simulink model "OPENXWD"  (R2021b)
settings: Solver=ode45  StartTime=0.0  StopTime=inf  RelTol=1e-3  EnableMultiTasking=on
PreLoadFcn:
  | run('Parameters\FSE_Parameters.m')
undefined symbols (not defined in the file): i_Diff
libraries: simulink x28, CarMaker4SL x17, eeGeneralControl x6
(part 2 of 8)

== system OPENXWD/CarMaker/IPG Vehicle/CarAndTrailer/Forces/Tires ==
  note: The TireXX_Out signals will only be used if FileIdent is "CarMaker-Tire-CM4SL" in the tire parameter file!
      | An example parameter file can be found in Data/Tire/DT_CM4SL_UserTire.
  Sync_In : Inport
  TireFL_In : Inport  Port=2
  TireFR_In : Inport  Port=3
  TireRL_In : Inport  Port=4
  TireRR_In : Inport  Port=5
  Bus Creator{1..4} (4 alike) : BusCreator  Inputs=11
  Demux{1..3,8} (4 alike) : Demux  Outputs=7
      settings: DisplayOption=none
  TireFL : Subsystem
  TireFR : Subsystem
  TireRL : Subsystem
  TireRR : Subsystem
  TireFL_Out : Outport
  TireFR_Out : Outport  Port=2
  TireRL_Out : Outport  Port=3
  TireRR_Out : Outport  Port=4
  wires:
  Sync_In/1 -> TireRR/1(Sync_In), TireRL/1(Sync_In), TireFR/1(Sync_In), TireFL/1(Sync_In)
  Bus Creator4/1 -> TireRR_Out/1
  Bus Creator2/1 -> TireRL_Out/1
  Bus Creator1/1 -> TireFR_Out/1
  Demux3/5 -> TireRR/6(Rim_turnv)  "Tire_In Rim_turnv"
  Demux3/4 -> TireRR/5(Rim_rotv)  "Tire_In Rim_rotv"
  Demux3/1 -> TireRR/2(Load)  "Tire_In Load"
  Demux3/7 -> TireRR/8(muRoad)  "Tire_In mu"
  Demux3/6 -> TireRR/7(InclinAngle)  "Tire_In Camber"
  Demux3/2 -> TireRR/3(vxtrans)  "Tire_In vxtrans"
  Demux3/3 -> TireRR/4(vytrans)  "Tire_In vytrans"
  TireRR/11(AlignTrq) -> Bus Creator4/11  "Tire_Out AlignTrq"
  TireRR/10(RollResist) -> Bus Creator4/10  "Tire_Out RollResist"
  TireRR/9(OverturnTrq) -> Bus Creator4/9  "Tire_Out OverturnTrq"
  TireRR/8(LoadFrc) -> Bus Creator4/8  "Tire_Out LoadFrc"
  TireRR/7(SideFrc) -> Bus Creator4/7  "Tire_Out SideFrc"
  TireRR/6(LongFrc) -> Bus Creator4/6  "Tire_Out LongFrc"
  TireRR/5(vBelt) -> Bus Creator4/5  "Tire_Out vBelt"
  TireRR/4(rBelt_eff) -> Bus Creator4/4  "Tire_Out rBelt_eff"
  TireRR/3(TurnSlp) -> Bus Creator4/3  "Tire_Out TurnSlp"
  TireRR/1(Slp) -> Bus Creator4/1  "Tire_Out Slp"
  TireRR/2(Alpha) -> Bus Creator4/2  "Tire_Out Alpha"
  Demux2/5 -> TireRL/6(Rim_turnv)  "Tire_In Rim_turnv"
  Demux2/4 -> TireRL/5(Rim_rotv)  "Tire_In Rim_rotv"
  Demux2/1 -> TireRL/2(Load)  "Tire_In Load"
  Demux2/7 -> TireRL/8(muRoad)  "Tire_In mu"
  Demux2/6 -> TireRL/7(InclinAngle)  "Tire_In Camber"
  Demux2/2 -> TireRL/3(vxtrans)  "Tire_In vxtrans"
  Demux2/3 -> TireRL/4(vytrans)  "Tire_In vytrans"
  TireRL/11(AlignTrq) -> Bus Creator2/11  "Tire_Out AlignTrq"
  TireRL/10(RollResist) -> Bus Creator2/10  "Tire_Out RollResist"
  TireRL/9(OverturnTrq) -> Bus Creator2/9  "Tire_Out OverturnTrq"
  TireRL/8(LoadFrc) -> Bus Creator2/8  "Tire_Out LoadFrc"
  TireRL/7(SideFrc) -> Bus Creator2/7  "Tire_Out SideFrc"
  TireRL/6(LongFrc) -> Bus Creator2/6  "Tire_Out LongFrc"
  TireRL/5(vBelt) -> Bus Creator2/5  "Tire_Out vBelt"
  TireRL/4(rBelt_eff) -> Bus Creator2/4  "Tire_Out rBelt_eff"
  TireRL/3(TurnSlp) -> Bus Creator2/3  "Tire_Out TurnSlp"
  TireRL/1(Slp) -> Bus Creator2/1  "Tire_Out Slp"
  TireRL/2(Alpha) -> Bus Creator2/2  "Tire_Out Alpha"
  Demux1/5 -> TireFR/6(Rim_turnv)  "Tire_In Rim_turnv"
  Demux1/4 -> TireFR/5(Rim_rotv)  "Tire_In Rim_rotv"
  Demux1/1 -> TireFR/2(Load)  "Tire_In Load"
  Demux1/7 -> TireFR/8(muRoad)  "Tire_In mu"
  Demux1/6 -> TireFR/7(InclinAngle)  "Tire_In Camber"
  Demux1/2 -> TireFR/3(vxtrans)  "Tire_In vxtrans"
  Demux1/3 -> TireFR/4(vytrans)  "Tire_In vytrans"
  TireFR/11(AlignTrq) -> Bus Creator1/11  "Tire_Out AlignTrq"
  TireFR/10(RollResist) -> Bus Creator1/10  "Tire_Out RollResist"
  TireFR/9(OverturnTrq) -> Bus Creator1/9  "Tire_Out OverturnTrq"
  TireFR/8(LoadFrc) -> Bus Creator1/8  "Tire_Out LoadFrc"
  TireFR/7(SideFrc) -> Bus Creator1/7  "Tire_Out SideFrc"
  TireFR/6(LongFrc) -> Bus Creator1/6  "Tire_Out LongFrc"
  TireFR/5(vBelt) -> Bus Creator1/5  "Tire_Out vBelt"
  TireFR/4(rBelt_eff) -> Bus Creator1/4  "Tire_Out rBelt_eff"
  TireFR/3(TurnSlp) -> Bus Creator1/3  "Tire_Out TurnSlp"
  TireFR/1(Slp) -> Bus Creator1/1  "Tire_Out Slp"
  TireFR/2(Alpha) -> Bus Creator1/2  "Tire_Out Alpha"
  Demux8/5 -> TireFL/6(Rim_turnv)  "Tire_In Rim_turnv"
  Demux8/4 -> TireFL/5(Rim_rotv)  "Tire_In Rim_rotv"
  TireFL_In/1 -> Demux8/1
  Demux8/1 -> TireFL/2(Load)  "Tire_In Load"
  Demux8/7 -> TireFL/8(muRoad)  "Tire_In mu"
  Demux8/6 -> TireFL/7(InclinAngle)  "Tire_In Camber"
  Demux8/2 -> TireFL/3(vxtrans)  "Tire_In vxtrans"
  Demux8/3 -> TireFL/4(vytrans)  "Tire_In vytrans"
  TireFL/11(AlignTrq) -> Bus Creator3/11  "Tire_Out AlignTrq"
  TireFL/10(RollResist) -> Bus Creator3/10  "Tire_Out RollResist"
  TireFL/9(OverturnTrq) -> Bus Creator3/9  "Tire_Out OverturnTrq"
  TireFL/8(LoadFrc) -> Bus Creator3/8  "Tire_Out LoadFrc"
  TireFL/7(SideFrc) -> Bus Creator3/7  "Tire_Out SideFrc"
  TireFL/6(LongFrc) -> Bus Creator3/6  "Tire_Out LongFrc"
  TireFL/5(vBelt) -> Bus Creator3/5  "Tire_Out vBelt"
  TireFL/4(rBelt_eff) -> Bus Creator3/4  "Tire_Out rBelt_eff"
  TireFL/3(TurnSlp) -> Bus Creator3/3  "Tire_Out TurnSlp"
  TireFL/1(Slp) -> Bus Creator3/1  "Tire_Out Slp"
  TireFL/2(Alpha) -> Bus Creator3/2  "Tire_Out Alpha"
  Bus Creator3/1 -> TireFL_Out/1
  TireFR_In/1 -> Demux1/1
  TireRL_In/1 -> Demux2/1
  TireRR_In/1 -> Demux3/1

== system OPENXWD/CarMaker/IPG Vehicle/CarAndTrailer/Forces/Vehicle Forces ==
  Sync_In : Inport
  Bus Creator1 : BusCreator  Inputs=12
  Bus Creator8 : BusCreator  Inputs=16
  BusCreator1 : BusCreator  Inputs=4
  BusCreator2 : BusCreator  Inputs=9
  Demux : Demux  Outputs=16
      settings: DisplayOption=none
  Demux1 : Demux  Outputs=12
      settings: DisplayOption=none
  Demux2 : Demux  Outputs=13
      settings: DisplayOption=none
  Forces : S-Function  FunctionName=CM_Sfun  Parameters='Forces'  SFunctionDeploymentMode=off  EnableBusSupport=off
  Terminator : Terminator
  Sync_Out : Outport
  Car.Virtual : Outport  Port=2
  Car.Aero : Outport  Port=3
  Car.Load : Outport  Port=4
  wires:
  BusCreator1/1 -> Terminator/1  "Aero IF (in)"
  Demux2/13 -> BusCreator2/9  "car Aero Trq_1 z"
  Demux2/12 -> BusCreator2/8  "car Aero Trq_1 y"
  Demux2/11 -> BusCreator2/7  "car Aero Trq_1 x"
  Demux2/10 -> BusCreator2/6  "car Aero Frc_1 z"
  Demux2/9 -> BusCreator2/5  "car Aero Frc_1 y"
  Demux2/8 -> BusCreator2/4  "car Aero Frc_1 x"
  Demux2/7 -> BusCreator2/3  "car Aero PoA_1 z"
  Demux2/6 -> BusCreator2/2  "car Aero PoA_1 y"
  Demux2/5 -> BusCreator2/1  "car Aero PoA_1 x"
  Demux2/4 -> BusCreator1/4  "car Aero tau_1"
  Demux2/3 -> BusCreator1/3  "car Aero ApproachVel_1 z"
  Demux2/2 -> BusCreator1/2  "car Aero ApproachVel_1 y"
  Demux2/1 -> BusCreator1/1  "car Aero ApproachVel_1 x"
  Demux/16 -> Bus Creator8/16  "Car Load_3 tz"
  Demux/15 -> Bus Creator8/15  "Car Load_3 ty"
  Demux/14 -> Bus Creator8/14  "Car Load_3 tx"
  Demux/13 -> Bus Creator8/13  "Car Load_3 mass"
  Demux1/12 -> Bus Creator1/12  "Car Virtual Trq_0 z"
  Demux1/11 -> Bus Creator1/11  "Car Virtual Trq_0 y"
  Demux1/10 -> Bus Creator1/10  "Car Virtual Trq_0 x"
  Demux1/9 -> Bus Creator1/9  "Car Virtual Trq_1 z"
  Demux1/8 -> Bus Creator1/8  "Car Virtual Trq_1 y"
  Demux1/7 -> Bus Creator1/7  "Car Virtual Trq_1 x"
  Demux1/6 -> Bus Creator1/6  "Car Virtual Frc_0 z"
  Demux1/5 -> Bus Creator1/5  "Car Virtual Frc_0 y"
  Demux1/4 -> Bus Creator1/4  "Car Virtual Frc_0 x"
  Sync_In/1 -> Forces/1
  Forces/1 -> Sync_Out/1
  BusCreator2/1 -> Car.Aero/1
  Demux1/1 -> Bus Creator1/1  "Car Virtual Frc_1 x"
  Demux1/2 -> Bus Creator1/2  "Car Virtual Frc_1 y"
  Demux1/3 -> Bus Creator1/3  "Car Virtual Frc_1 z"
  Forces/3 -> Demux2/1
  Forces/2 -> Demux1/1
  Bus Creator1/1 -> Car.Virtual/1
  Bus Creator8/1 -> Car.Load/1
  Demux/1 -> Bus Creator8/1  "Car Load_0 mass"
  Demux/2 -> Bus Creator8/2  "Car Load_0 tx"
  Demux/3 -> Bus Creator8/3  "Car Load_0 ty"
  Demux/4 -> Bus Creator8/4  "Car Load_0 tz"
  Demux/5 -> Bus Creator8/5  "Car Load_1 mass"
  Demux/6 -> Bus Creator8/6  "Car Load_1 tx"
  Demux/7 -> Bus Creator8/7  "Car Load_1 ty"
  Demux/8 -> Bus Creator8/8  "Car Load_1 tz"
  Demux/9 -> Bus Creator8/9  "Car Load_2 mass"
  Demux/10 -> Bus Creator8/10  "Car Load_2 tx"
  Demux/11 -> Bus Creator8/11  "Car Load_2 ty"
  Demux/12 -> Bus Creator8/12  "Car Load_2 tz"
  Forces/4 -> Demux/1

== system OPENXWD/CarMaker/IPG Vehicle/CarAndTrailer/Trailer/CreateBus Car.Hitch.FrcTrq ==
  In1 : Inport
  Bus Creator7 : BusCreator  Inputs=6
  Demux7 : Demux  Outputs=6
      settings: DisplayOption=none
  Out1 : Outport
  wires:
  In1/1 -> Demux7/1
  Bus Creator7/1 -> Out1/1
  Demux7/6 -> Bus Creator7/6  "Car Hitch Trq2Car z"
  Demux7/5 -> Bus Creator7/5  "Car Hitch Trq2Car y"
  Demux7/4 -> Bus Creator7/4  "Car Hitch Trq2Car x"
  Demux7/3 -> Bus Creator7/3  "Car Hitch Frc2Car z"
  Demux7/2 -> Bus Creator7/2  "Car Hitch Frc2Car y"
  Demux7/1 -> Bus Creator7/1  "Car Hitch Frc2Car x"

== system OPENXWD/CarMaker/IPG Vehicle/CarAndTrailer/Trailer/CreateBus Vhcl.Motion ==
  In1 : Inport
  BusCreator : BusCreator  Inputs=15
  Demux : Demux  Outputs=15
      settings: DisplayOption=none
  Out1 : Outport
  wires:
  Demux/15 -> BusCreator/15  "Vhcl YawAcc"
  Demux/14 -> BusCreator/14  "Vhcl YawVel"
  Demux/13 -> BusCreator/13  "Vhcl Yaw"
  Demux/12 -> BusCreator/12  "Vhcl PitchAcc"
  Demux/11 -> BusCreator/11  "Vhcl PitchVel"
  Demux/10 -> BusCreator/10  "Vhcl Pitch"
  Demux/9 -> BusCreator/9  "Vhcl RollAcc"
  Demux/8 -> BusCreator/8  "Vhcl RollVel"
  Demux/7 -> BusCreator/7  "Vhcl Roll"
  Demux/6 -> BusCreator/6  "Vhcl Hitch_Pos z"
  Demux/5 -> BusCreator/5  "Vhcl Hitch_Pos y"
  Demux/4 -> BusCreator/4  "Vhcl Hitch_Pos x"
  Demux/3 -> BusCreator/3  "Vhcl sRoad"
  Demux/2 -> BusCreator/2  "Vhcl Distance"
  Demux/1 -> BusCreator/1  "Vhcl v"
  In1/1 -> Demux/1
  BusCreator/1 -> Out1/1

== system OPENXWD/CarMaker/IPG Vehicle/CarAndTrailer/Trailer/CreateBus Vhcl.PoI ==
  In1 : Inport
  Bus Creator3 : BusCreator  Inputs=18
  Demux3 : Demux  Outputs=18
      settings: DisplayOption=none
  Out1 : Outport
  wires:
  Demux3/18 -> Bus Creator3/18  "Vhcl PoI_GCS Elev"
  Demux3/17 -> Bus Creator3/17  "Vhcl PoI_GCS Lat"
  Demux3/16 -> Bus Creator3/16  "Vhcl PoI_GCS Long"
  Demux3/15 -> Bus Creator3/15  "Vhcl PoI_Acc_1 z"
  Demux3/14 -> Bus Creator3/14  "Vhcl PoI_Acc_1 y"
  Demux3/13 -> Bus Creator3/13  "Vhcl PoI_Acc_1 x"
  Demux3/12 -> Bus Creator3/12  "Vhcl PoI_Vel_1 z"
  Demux3/11 -> Bus Creator3/11  "Vhcl PoI_Vel_1 y"
  Demux3/10 -> Bus Creator3/10  "Vhcl PoI_Vel_1 x"
  Demux3/9 -> Bus Creator3/9  "Vhcl PoI_Acc z"
  Demux3/8 -> Bus Creator3/8  "Vhcl PoI_Acc y"
  Demux3/7 -> Bus Creator3/7  "Vhcl PoI_Acc x"
  Demux3/6 -> Bus Creator3/6  "Vhcl PoI_Vel z"
  Demux3/5 -> Bus Creator3/5  "Vhcl PoI_Vel y"
  Demux3/4 -> Bus Creator3/4  "Vhcl PoI_Vel x"
  Demux3/3 -> Bus Creator3/3  "Vhcl PoI_Pos z"
  Demux3/2 -> Bus Creator3/2  "Vhcl PoI_Pos y"
  In1/1 -> Demux3/1
  Bus Creator3/1 -> Out1/1
  Demux3/1 -> Bus Creator3/1  "Vhcl PoI_Pos x"

== system OPENXWD/CarMaker/IPG Vehicle/CarAndTrailer/Trailer/CreateBus Vhcl.Steering ==
  In1 : Inport
  Bus Creator3 : BusCreator  Inputs=4
  Demux : Demux
      settings: DisplayOption=none
  Out1 : Outport
  wires:
  Bus Creator3/1 -> Out1/1
  Demux/1 -> Bus Creator3/1  "Vhcl Steering Ang"
  Demux/3 -> Bus Creator3/3  "Vhcl Steering AngAcc"
  Demux/2 -> Bus Creator3/2  "Vhcl Steering AngVel"
  Demux/4 -> Bus Creator3/4  "Vhcl Steering Trq"
  In1/1 -> Demux/1

== system OPENXWD/CarMaker/IPG Vehicle/CarAndTrailer/Trailer/CreateBus Vhcl.Wheel.FL ==
  In1 : Inport
  Bus Creator3 : BusCreator  Inputs=14
  Demux3 : Demux  Outputs=14
      settings: DisplayOption=none
  Out1 : Outport
  wires:
  Demux3/14 -> Bus Creator3/14  "Vhcl Wheel FL Trq_WhlBearing"
  Demux3/13 -> Bus Creator3/13  "Vhcl Wheel FL Trq_T2W"
  Demux3/12 -> Bus Creator3/12  "Vhcl Wheel FL SideSlip"
  Demux3/11 -> Bus Creator3/11  "Vhcl Wheel FL LongSlip"
  Demux3/10 -> Bus Creator3/10  "Vhcl Wheel FL vBelt"
  Demux3/9 -> Bus Creator3/9  "Vhcl Wheel FL Fz"
  Demux3/8 -> Bus Creator3/8  "Vhcl Wheel FL Fy"
  Demux3/7 -> Bus Creator3/7  "Vhcl Wheel FL Fx"
  Demux3/6 -> Bus Creator3/6  "Vhcl Wheel FL r_zxy z"
  Demux3/5 -> Bus Creator3/5  "Vhcl Wheel FL r_zxy y"
  Demux3/4 -> Bus Creator3/4  "Vhcl Wheel FL r_zxy x"
  Demux3/3 -> Bus Creator3/3  "Vhcl Wheel FL t z"
  Demux3/2 -> Bus Creator3/2  "Vhcl Wheel FL t y"
  In1/1 -> Demux3/1
  Bus Creator3/1 -> Out1/1
  Demux3/1 -> Bus Creator3/1  "Vhcl Wheel FL t x"

== system OPENXWD/CarMaker/IPG Vehicle/CarAndTrailer/Trailer/CreateBus Vhcl.Wheel.FR ==
  In1 : Inport
  Bus Creator3 : BusCreator  Inputs=14
  Demux3 : Demux  Outputs=14
      settings: DisplayOption=none
  Out1 : Outport
  wires:
  Demux3/14 -> Bus Creator3/14  "Vhcl Wheel FR Trq_WhlBearing"
  Demux3/13 -> Bus Creator3/13  "Vhcl Wheel FR Trq_T2W"
  Demux3/12 -> Bus Creator3/12  "Vhcl Wheel FR SideSlip"
  Demux3/11 -> Bus Creator3/11  "Vhcl Wheel FR LongSlip"
  Demux3/10 -> Bus Creator3/10  "Vhcl Wheel FR vBelt"
  Demux3/9 -> Bus Creator3/9  "Vhcl Wheel FR Fz"
  Demux3/8 -> Bus Creator3/8  "Vhcl Wheel FR Fy"
  Demux3/7 -> Bus Creator3/7  "Vhcl Wheel FR Fx"
  Demux3/6 -> Bus Creator3/6  "Vhcl Wheel FR r_zxy z"
  Demux3/5 -> Bus Creator3/5  "Vhcl Wheel FR r_zxy y"
  Demux3/4 -> Bus Creator3/4  "Vhcl Wheel FR r_zxy x"
  Demux3/3 -> Bus Creator3/3  "Vhcl Wheel FR t z"
  Demux3/2 -> Bus Creator3/2  "Vhcl Wheel FR t y"
  In1/1 -> Demux3/1
  Bus Creator3/1 -> Out1/1
  Demux3/1 -> Bus Creator3/1  "Vhcl Wheel FR t x"

== system OPENXWD/CarMaker/IPG Vehicle/CarAndTrailer/Trailer/CreateBus Vhcl.Wheel.RL ==
  In1 : Inport
  Bus Creator3 : BusCreator  Inputs=14
  Demux3 : Demux  Outputs=14
      settings: DisplayOption=none
  Out1 : Outport
  wires:
  Demux3/14 -> Bus Creator3/14  "Vhcl Wheel RL Trq_WhlBearing"
  Demux3/13 -> Bus Creator3/13  "Vhcl Wheel RL Trq_T2W"
  Demux3/12 -> Bus Creator3/12  "Vhcl Wheel RL SideSlip"
  Demux3/11 -> Bus Creator3/11  "Vhcl Wheel RL LongSlip"
  Demux3/10 -> Bus Creator3/10  "Vhcl Wheel RL vBelt"
  Demux3/9 -> Bus Creator3/9  "Vhcl Wheel RL Fz"
  Demux3/8 -> Bus Creator3/8  "Vhcl Wheel RL Fy"
  Demux3/7 -> Bus Creator3/7  "Vhcl Wheel RL Fx"
  Demux3/6 -> Bus Creator3/6  "Vhcl Wheel RL r_zxy z"
  Demux3/5 -> Bus Creator3/5  "Vhcl Wheel RL r_zxy y"
  Demux3/4 -> Bus Creator3/4  "Vhcl Wheel RL r_zxy x"
  Demux3/3 -> Bus Creator3/3  "Vhcl Wheel RL t z"
  Demux3/2 -> Bus Creator3/2  "Vhcl Wheel RL t y"
  In1/1 -> Demux3/1
  Bus Creator3/1 -> Out1/1
  Demux3/1 -> Bus Creator3/1  "Vhcl Wheel RL t x"

== system OPENXWD/CarMaker/IPG Vehicle/CarAndTrailer/Trailer/CreateBus Vhcl.Wheel.RR ==
  In1 : Inport
  Bus Creator3 : BusCreator  Inputs=14
  Demux3 : Demux  Outputs=14
      settings: DisplayOption=none
  Out1 : Outport
  wires:
  Demux3/14 -> Bus Creator3/14  "Vhcl Wheel RR Trq_WhlBearing"
  Demux3/13 -> Bus Creator3/13  "Vhcl Wheel RR Trq_T2W"
  Demux3/12 -> Bus Creator3/12  "Vhcl Wheel RR SideSlip"
  Demux3/11 -> Bus Creator3/11  "Vhcl Wheel RR LongSlip"
  Demux3/10 -> Bus Creator3/10  "Vhcl Wheel RR vBelt"
  Demux3/9 -> Bus Creator3/9  "Vhcl Wheel RR Fz"
  Demux3/8 -> Bus Creator3/8  "Vhcl Wheel RR Fy"
  Demux3/7 -> Bus Creator3/7  "Vhcl Wheel RR Fx"
  Demux3/6 -> Bus Creator3/6  "Vhcl Wheel RR r_zxy z"
  Demux3/5 -> Bus Creator3/5  "Vhcl Wheel RR r_zxy y"
  Demux3/4 -> Bus Creator3/4  "Vhcl Wheel RR r_zxy x"
  Demux3/3 -> Bus Creator3/3  "Vhcl Wheel RR t z"
  Demux3/2 -> Bus Creator3/2  "Vhcl Wheel RR t y"
  In1/1 -> Demux3/1
  Bus Creator3/1 -> Out1/1
  Demux3/1 -> Bus Creator3/1  "Vhcl Wheel RR t x"

== system OPENXWD/CarMaker/IPG Vehicle/PowerTrain/Electric Powertrain/E-Gas // E-Motor ==
  VhclCtrl.Brake : Inport
  VC.Gas : Inport  Port=2
  VhclCtrl.Steering : Inport  Port=3
  Bus Selector : BusSelector  OutputSignals=VhclCtrl Brake
  Bus Selector1 : BusSelector  OutputSignals=VhclCtrl Steering Ang
  Constant14 : Constant  Value=3
  Rad to º : Gain  Gain=180/3.141593
  Read CM Dict : CarMaker4SL/Read CM Dict  xname=Car.WheelSpd_RL  xsync=off  xstime=Continuous
  Read CM Dict1 : CarMaker4SL/Read CM Dict  xname=Car.WheelSpd_RR  xsync=off  xstime=Continuous
  Read CM Dict2 : CarMaker4SL/Read CM Dict  xname=Car.FzRR  xsync=off  xstime=Continuous
  Read CM Dict3 : CarMaker4SL/Read CM Dict  xname=Car.FzRL  xsync=off  xstime=Continuous
  Read CM Dict4 : CarMaker4SL/Read CM Dict  xname=Car.vxRR  xsync=off  xstime=Continuous
  Read CM Dict5 : CarMaker4SL/Read CM Dict  xname=Car.vxRL  xsync=off  xstime=Continuous
  Read CM Dict6 : CarMaker4SL/Read CM Dict  xname=Car.FzFL  xsync=off  xstime=Continuous
  Read CM Dict7 : CarMaker4SL/Read CM Dict  xname=Car.FzFR  xsync=off  xstime=Continuous
  Read CM Dict8 : CarMaker4SL/Read CM Dict  xname=Car.ay  xsync=off  xstime=Continuous
  Subsystem : Subsystem
  m/s to km/h : Gain  Gain=3.6
  m/s to km/h1 : Gain  Gain=3.6
  Trq_RL : Outport  VectorParamsAs1DForOutWhenUnconnected=off
  Trq_RR : Outport  Port=2  VectorParamsAs1DForOutWhenUnconnected=off
  wires:
  VC.Gas/1 -> Subsystem/27(APPS1_Value), Subsystem/26(APPS2_Value)
  VhclCtrl.Brake/1 -> Bus Selector/1
  VhclCtrl.Steering/1 -> Bus Selector1/1
  Bus Selector/1 -> Subsystem/28(BrakeSensor_Value)  "<VhclCtrl Brake>"
  Subsystem/29(Torque_L) -> Trq_RL/1
  Subsystem/30(Torque_R) -> Trq_RR/1
  Read CM Dict1/1 -> Subsystem/36(RR_rads)
  Read CM Dict/1 -> Subsystem/35(RL_rads)
  Read CM Dict3/1 -> Subsystem/31(Susp_R_L)
  Read CM Dict2/1 -> Subsystem/32(Susp_R_R)
  Read CM Dict4/1 -> m/s to km/h/1
  Read CM Dict5/1 -> m/s to km/h1/1
  m/s to km/h/1 -> Subsystem/33(Vel_RL_kmh)
  m/s to km/h1/1 -> Subsystem/34(Vel_RR_kmh)
  Read CM Dict6/1 -> Subsystem/29(Susp_F_L)
  Read CM Dict7/1 -> Subsystem/30(Susp_F_R)
  Constant14/1 -> Subsystem/13(TV_Mode)
  Read CM Dict8/1 -> Subsystem/19(ACCEL_R_Y_SI)
  Bus Selector1/1 -> Rad to º/1  "<VhclCtrl Steering Ang>"
  Rad to º/1 -> Subsystem/14(SteeringSensor)

== system OPENXWD/CarMaker/IPG Vehicle/PowerTrain/Electric Powertrain/Gas Pedal ==
  Clock : Clock
  Constant : Constant  Value=0
  Constant1 : Constant
  Fcn : Fcn  Expr=u==0
  Read CM Dict : CarMaker4SL/Read CM Dict  xname=Vhcl.Ignition  xsync=off  xstime=Continuous
  Read CM Dict2 : CarMaker4SL/Read CM Dict  xname=VC.Gas  xsync=off  xstime=Continuous
  Switch : Switch
  Switch1 : Switch
  Write CM Dict : CarMaker4SL/Write CM Dict  xname=Vhcl.Ignition  xsync=off
  VC.Gas : Outport  VectorParamsAs1DForOutWhenUnconnected=off
  wires:
  Read CM Dict2/1 -> Switch/1
  Switch/1 -> VC.Gas/1
  Constant/1 -> Switch/3
  Switch1/1 -> Switch/2, Write CM Dict/1
  Read CM Dict/1 -> Switch1/3
  Constant1/1 -> Switch1/1
  Fcn/1 -> Switch1/2
  Clock/1 -> Fcn/1

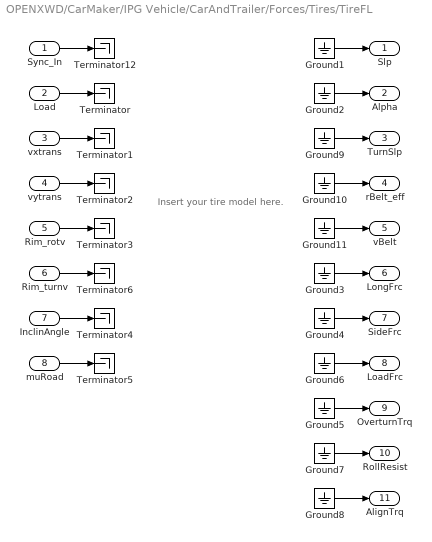
== system OPENXWD/CarMaker/IPG Vehicle/CarAndTrailer/Forces/Tires/TireFL ==
  note: Insert your tire model here.
  Sync_In : Inport
  Load : Inport  Port=2
  vxtrans : Inport  Port=3
  vytrans : Inport  Port=4
  Rim_rotv : Inport  Port=5
  Rim_turnv : Inport  Port=6
  InclinAngle : Inport  Port=7
  muRoad : Inport  Port=8
  Ground{1..11} (11 alike) : Ground
  Terminator{,1..6,12} (8 alike) : Terminator
  Slp : Outport
  Alpha : Outport  Port=2
  TurnSlp : Outport  Port=3
  rBelt_eff : Outport  Port=4
  vBelt : Outport  Port=5
  LongFrc : Outport  Port=6
  SideFrc : Outport  Port=7
  LoadFrc : Outport  Port=8
  OverturnTrq : Outport  Port=9
  RollResist : Outport  Port=10
  AlignTrq : Outport  Port=11
  wires:
  Ground11/1 -> vBelt/1
  Ground10/1 -> rBelt_eff/1
  Ground9/1 -> TurnSlp/1
  Rim_turnv/1 -> Terminator6/1
  Sync_In/1 -> Terminator12/1
  Ground2/1 -> Alpha/1
  Ground3/1 -> LongFrc/1
  Ground4/1 -> SideFrc/1
  Ground5/1 -> OverturnTrq/1
  vxtrans/1 -> Terminator1/1
  vytrans/1 -> Terminator2/1
  Rim_rotv/1 -> Terminator3/1
  InclinAngle/1 -> Terminator4/1
  muRoad/1 -> Terminator5/1
  Load/1 -> Terminator/1
  Ground1/1 -> Slp/1
  Ground6/1 -> LoadFrc/1
  Ground7/1 -> RollResist/1
  Ground8/1 -> AlignTrq/1

== system OPENXWD/CarMaker/IPG Vehicle/CarAndTrailer/Forces/Tires/TireFR ==
  note: Insert your tire model here.
  Sync_In : Inport
  Load : Inport  Port=2
  vxtrans : Inport  Port=3
  vytrans : Inport  Port=4
  Rim_rotv : Inport  Port=5
  Rim_turnv : Inport  Port=6
  InclinAngle : Inport  Port=7
  muRoad : Inport  Port=8
  Ground{1..11} (11 alike) : Ground
  Terminator{,1..6,12} (8 alike) : Terminator
  Slp : Outport
  Alpha : Outport  Port=2
  TurnSlp : Outport  Port=3
  rBelt_eff : Outport  Port=4
  vBelt : Outport  Port=5
  LongFrc : Outport  Port=6
  SideFrc : Outport  Port=7
  LoadFrc : Outport  Port=8
  OverturnTrq : Outport  Port=9
  RollResist : Outport  Port=10
  AlignTrq : Outport  Port=11
  wires:
  Ground11/1 -> vBelt/1
  Ground10/1 -> rBelt_eff/1
  Ground9/1 -> TurnSlp/1
  Rim_turnv/1 -> Terminator6/1
  Sync_In/1 -> Terminator12/1
  Ground2/1 -> Alpha/1
  Ground3/1 -> LongFrc/1
  Ground4/1 -> SideFrc/1
  Ground5/1 -> OverturnTrq/1
  vxtrans/1 -> Terminator1/1
  vytrans/1 -> Terminator2/1
  Rim_rotv/1 -> Terminator3/1
  InclinAngle/1 -> Terminator4/1
  muRoad/1 -> Terminator5/1
  Load/1 -> Terminator/1
  Ground1/1 -> Slp/1
  Ground6/1 -> LoadFrc/1
  Ground7/1 -> RollResist/1
  Ground8/1 -> AlignTrq/1

== system OPENXWD/CarMaker/IPG Vehicle/CarAndTrailer/Forces/Tires/TireRL ==
  note: Insert your tire model here.
  Sync_In : Inport
  Load : Inport  Port=2
  vxtrans : Inport  Port=3
  vytrans : Inport  Port=4
  Rim_rotv : Inport  Port=5
  Rim_turnv : Inport  Port=6
  InclinAngle : Inport  Port=7
  muRoad : Inport  Port=8
  Ground{1..11} (11 alike) : Ground
  Terminator{,1..6,12} (8 alike) : Terminator
  Slp : Outport
  Alpha : Outport  Port=2
  TurnSlp : Outport  Port=3
  rBelt_eff : Outport  Port=4
  vBelt : Outport  Port=5
  LongFrc : Outport  Port=6
  SideFrc : Outport  Port=7
  LoadFrc : Outport  Port=8
  OverturnTrq : Outport  Port=9
  RollResist : Outport  Port=10
  AlignTrq : Outport  Port=11
  wires:
  Ground11/1 -> vBelt/1
  Ground10/1 -> rBelt_eff/1
  Ground9/1 -> TurnSlp/1
  Rim_turnv/1 -> Terminator6/1
  Sync_In/1 -> Terminator12/1
  Ground2/1 -> Alpha/1
  Ground3/1 -> LongFrc/1
  Ground4/1 -> SideFrc/1
  Ground5/1 -> OverturnTrq/1
  vxtrans/1 -> Terminator1/1
  vytrans/1 -> Terminator2/1
  Rim_rotv/1 -> Terminator3/1
  InclinAngle/1 -> Terminator4/1
  muRoad/1 -> Terminator5/1
  Load/1 -> Terminator/1
  Ground1/1 -> Slp/1
  Ground6/1 -> LoadFrc/1
  Ground7/1 -> RollResist/1
  Ground8/1 -> AlignTrq/1

== system OPENXWD/CarMaker/IPG Vehicle/CarAndTrailer/Forces/Tires/TireRR ==
  note: Insert your tire model here.
  Sync_In : Inport
  Load : Inport  Port=2
  vxtrans : Inport  Port=3
  vytrans : Inport  Port=4
  Rim_rotv : Inport  Port=5
  Rim_turnv : Inport  Port=6
  InclinAngle : Inport  Port=7
  muRoad : Inport  Port=8
  Ground{1..11} (11 alike) : Ground
  Terminator{,1..6,12} (8 alike) : Terminator
  Slp : Outport
  Alpha : Outport  Port=2
  TurnSlp : Outport  Port=3
  rBelt_eff : Outport  Port=4
  vBelt : Outport  Port=5
  LongFrc : Outport  Port=6
  SideFrc : Outport  Port=7
  LoadFrc : Outport  Port=8
  OverturnTrq : Outport  Port=9
  RollResist : Outport  Port=10
  AlignTrq : Outport  Port=11
  wires:
  Ground11/1 -> vBelt/1
  Ground10/1 -> rBelt_eff/1
  Ground9/1 -> TurnSlp/1
  Rim_turnv/1 -> Terminator6/1
  Sync_In/1 -> Terminator12/1
  Ground2/1 -> Alpha/1
  Ground3/1 -> LongFrc/1
  Ground4/1 -> SideFrc/1
  Ground5/1 -> OverturnTrq/1
  vxtrans/1 -> Terminator1/1
  vytrans/1 -> Terminator2/1
  Rim_rotv/1 -> Terminator3/1
  InclinAngle/1 -> Terminator4/1
  muRoad/1 -> Terminator5/1
  Load/1 -> Terminator/1
  Ground1/1 -> Slp/1
  Ground6/1 -> LoadFrc/1
  Ground7/1 -> RollResist/1
  Ground8/1 -> AlignTrq/1

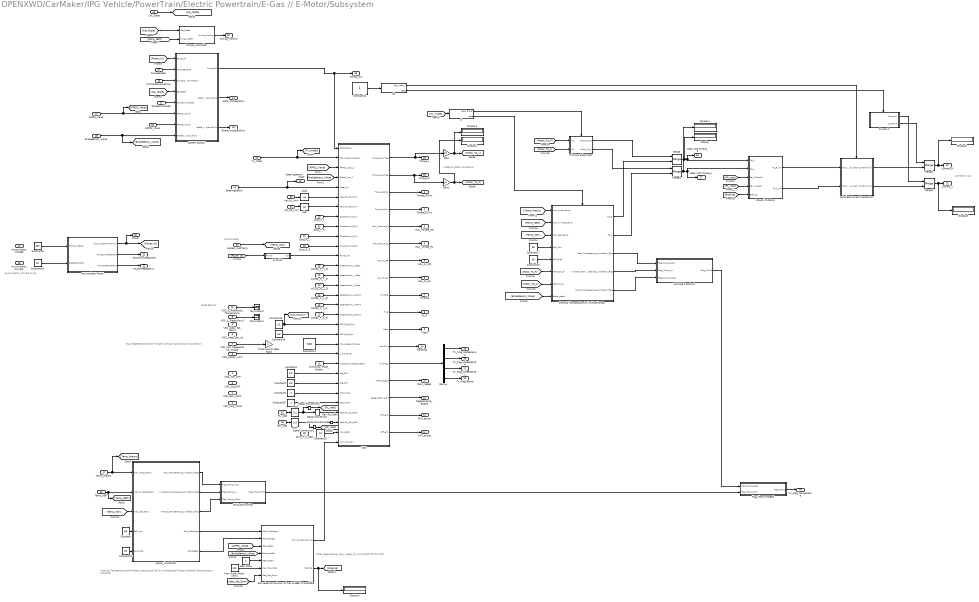
== system OPENXWD/CarMaker/IPG Vehicle/PowerTrain/Electric Powertrain/E-Gas // E-Motor/Subsystem ==
  note: When regenerating, Sum_wheel_Tq_max POSITIVE (for FM0)
  note: Accumulator
  note: Max Regenerative Motor Torque (without transmission convertion)
  note: Wheel to Motor conversion
  note: Accumulator_Current in [A]
  note: Controls Temperature and Protects because of SoC by limiting total Power available (discharging or charging)
  note: Mode Params
  note: currents in [A]
  VDC_SKF_Initial : Inport
  VDC_CKF_Initial : Inport  Port=2
  VDC_Cte_SKF : Inport  Port=3
  VDC_Cte_CKF : Inport  Port=4
  VDC_Apps_Sat_Down : Inport  Port=5
  VDC_Apps_Sat_Up : Inport  Port=6
  VDC_Max_Regenerative_Torque : Inport  Port=7
  VDC_Power_Limit : Inport  Port=8
  VDC_K_Reduction_P : Inport  Port=9
  VDC_K_Reduction_Temperature : Inport  Port=10
  Workshop_Mode_Enable : Inport  Port=11
  TorqueEnable : Inport  Port=12
  TV_Mode : Inport  Port=13
  SteeringSensor : Inport  Port=14
  Highest_CellTemp : Inport  Port=15
  CriticalDisconnection : Inport  Port=16
  ShutdownClosed : Inport  Port=17
  ACCEL_R_X_SI : Inport  Port=18
  ACCEL_R_Y_SI : Inport  Port=19
  ACCEL_R_Z_SI : Inport  Port=20
  ACCEL_F_X_SI : Inport  Port=21
  ACCEL_F_Y_SI : Inport  Port=22
  ACCEL_F_Z_SI : Inport  Port=23
  Accumulator_Voltage : Inport  Port=24
  Accumulator_Current : Inport  Port=25
  APPS2_Value : Inport  Port=26
  APPS1_Value : Inport  Port=27
  BrakeSensor_Value : Inport  Port=28
  Susp_F_L : Inport  Port=29
  Susp_F_R : Inport  Port=30
  Susp_R_L : Inport  Port=31
  Susp_R_R : Inport  Port=32
  Vel_RL_kmh : Inport  Port=33
  Vel_RR_kmh : Inport  Port=34
  RL_rads : Inport  Port=35
  RR_rads : Inport  Port=36
  Temp_Motors : Inport  Port=37
  Temp_IGBT : Inport  Port=38
  Gyro_F_Z_Deg : Inport  Port=39
  Car_State : Inport  Port=40
  Abs{,1..3} (4 alike) : Abs
  Accumulator Power : Subsystem
  Calculate Current Conversion : Subsystem
  Constant{,12..13,17} (4 alike) : Constant  Value=50
  Constant1 : Constant
  Constant10 : Constant  Value=20
  Constant11 : Constant  Value=500
  Constant18 : Constant  Value=0.2
  Constant19 : Constant  Value=0.8
  Constant2 : Constant  Value=0.9
  Constant20 : Constant
  Constant21 : Constant
  Constant23 : Constant  Value=10
  Constant3 : Constant  Value=0.9
  Constant9 : Constant  Value=400
  Controls Temperature by limiting Torque : Subsystem  TreatAsAtomicUnit=on
  Current 0 : Subsystem  TreatAsAtomicUnit=on
  Demux : Demux
  Display{,1..6} (7 alike) : Display
  Flag_Temp merged : MATLAB Function  TreatAsAtomicUnit=on
  Gain : Gain  Gain=1/4
  Gain1 : Gain  Gain=1/4
  Gear Ratio : Constant  Value=4
  If : If  IfExpression=u1 == 0
  If Action Subsystem : Subsystem  TreatAsAtomicUnit=on
  If1 : If  IfExpression=u1 == 1
  MATLAB Function : MATLAB Function  TreatAsAtomicUnit=on
  MATLAB Function1 : MATLAB Function  TreatAsAtomicUnit=on
  Max Tq per motor [Nm] : Constant  Value=120
  Merge{,1..3} (4 alike) : Merge
  Power limitation : Subsystem
  Pumps_Controller : Subsystem
  SAFETY BLOCK : Subsystem
  Signal Conversion{,1..3} (4 alike) : SignalConversion  OverrideOpt=off
  SoP selection and sum of max WHEEL Tq available : MATLAB Function  TreatAsAtomicUnit=on
  Terminator1 : Terminator
  Terminator2 : Terminator
  Transmission Gear Ratio : Gain  Gain=4
  VDC : Subsystem
  W to kW : Subsystem
  power_limitation1 : Subsystem
  Torque_RRwc : Outport  VectorParamsAs1DForOutWhenUnconnected=off
  Torque_RLwc : Outport  Port=2  VectorParamsAs1DForOutWhenUnconnected=off
  Max_Torque_RR : Outport  Port=3  VectorParamsAs1DForOutWhenUnconnected=off
  Max_Torque_RL : Outport  Port=4  VectorParamsAs1DForOutWhenUnconnected=off
  Max_Fx_RR : Outport  Port=5  VectorParamsAs1DForOutWhenUnconnected=off
  Max_Fx_RL : Outport  Port=6  VectorParamsAs1DForOutWhenUnconnected=off
  Throttle : Outport  Port=7  VectorParamsAs1DForOutWhenUnconnected=off
  Fy_R : Outport  Port=8  VectorParamsAs1DForOutWhenUnconnected=off
  Mass : Outport  Port=9  VectorParamsAs1DForOutWhenUnconnected=off
  Handling : Outport  Port=10  VectorParamsAs1DForOutWhenUnconnected=off
  SKF_actual : Outport  Port=11  VectorParamsAs1DForOutWhenUnconnected=off
  CKF_actual : Outport  Port=12  VectorParamsAs1DForOutWhenUnconnected=off
  SteeringSensor_Value : Outport  Port=13  VectorParamsAs1DForOutWhenUnconnected=off
  APPS_Implausibility : Outport  Port=14  VectorParamsAs1DForOutWhenUnconnected=off
  Brake_Implausibility : Outport  Port=15  VectorParamsAs1DForOutWhenUnconnected=off
  TV_Flag_WheelSpinRR : Outport  Port=16  VectorParamsAs1DForOutWhenUnconnected=off
  TV_Flag_WheelSpinRL : Outport  Port=17  VectorParamsAs1DForOutWhenUnconnected=off
  TV_Flag_Power : Outport  Port=18  VectorParamsAs1DForOutWhenUnconnected=off
  TV_Flag_CarBehaviour : Outport  Port=19  VectorParamsAs1DForOutWhenUnconnected=off
  Power : Outport  Port=20  VectorParamsAs1DForOutWhenUnconnected=off
  PowerLimitReached : Outport  Port=21  VectorParamsAs1DForOutWhenUnconnected=off
  PowerMean500ms : Outport  Port=22  VectorParamsAs1DForOutWhenUnconnected=off
  Torque_OK : Outport  Port=23  VectorParamsAs1DForOutWhenUnconnected=off
  Regenerative_Enable : Outport  Port=24  VectorParamsAs1DForOutWhenUnconnected=off
  Dash_Speed : Outport  Port=25  VectorParamsAs1DForOutWhenUnconnected=off
  Pumps_Control : Outport  Port=26  VectorParamsAs1DForOutWhenUnconnected=off
  Meas VDC Torque_L : Outport  Port=27  VectorParamsAs1DForOutWhenUnconnected=off
  Meas VDC Torque_R : Outport  Port=28  VectorParamsAs1DForOutWhenUnconnected=off
  Torque_L : Outport  Port=29  VectorParamsAs1DForOutWhenUnconnected=off
  Torque_R : Outport  Port=30  VectorParamsAs1DForOutWhenUnconnected=off
  current_L : Outport  Port=31  VectorParamsAs1DForOutWhenUnconnected=off
  current_R : Outport  Port=32  VectorParamsAs1DForOutWhenUnconnected=off
  TV_Flag_Temperature : Outport  Port=33  VectorParamsAs1DForOutWhenUnconnected=off
  wires:
  Accumulator Power/1(AccumulatorPower [W]) -> [Power_W], Power/1
  Constant1/1 -> VDC/26(SKF_Initial)
  Workshop_Mode_Enable/1 -> VDC/23(Workshop_Mode_Enable)
  power_limitation1/2(Inverters_Temperature_Limitation_Flag) -> MATLAB Function/2(Flag_Temp_Inv)
  [Temp_Cell] -> Controls Temperature by limiting Torque/3(max_cell_temp)
  [Power_W] -> SAFETY BLOCK/1(Power_W)
  [Temp_IGBT] -> Controls Temperature by limiting Torque/2(max_inverter_temp)
  Temp_Motors/1 -> power_limitation1/1(max_motor_temp), [Temp_Motors]
  Constant21/1 -> If1/1
  SAFETY BLOCK/2(APPS_Implausibility) -> APPS_Implausibility/1
  [Motor_Tq_L] -> If Action Subsystem/2(In2)
  [RR_rads] -> Power limitation/3(Rev_R [rads])
  Power limitation/1(Tq_R_lim) -> Calculate Current Conversion/1(Torque_R_motor)
  Controls Temperature by limiting Torque/5(Motors_Temperature_Limitation_Flag) -> MATLAB Function1/3(Flag_Temp_Motor)
  power_limitation1/1(Accu_Temperature_Limitation_Flag) -> MATLAB Function/1(Flag_Temp_Accu)
  Vel_RR_kmh/1 -> Abs/1
  [Braking] -> Power limitation/5(Braking)
  If1/2 -> Current 0/Action
  VDC/14(Mean_Speed) -> Dash_Speed/1
  ACCEL_F_Y_SI/1 -> VDC/17(Acceleration_Y_Front)
  APPS2_Value/1 -> SAFETY BLOCK/7(APPS2_Value)
  Flag_Temp merged/1(Flag_Temp) -> TV_Flag_Temperature/1
  [BrakeSensor_Value] -> VDC/4(Brake_0_to_1)
  SoP selection and sum of max WHEEL Tq available/2(Braking) -> Display4/1, [Braking]
  Current 0/1(Current L) -> Merge1/1
  [Apps_Sat_Down] -> SoP selection and sum of max WHEEL Tq available/7(Gas_Sat_Down)
  [Motor_Tq_R] -> If Action Subsystem/1(In1)
  Highest_CellTemp/1 -> [Temp_Cell]
  VDC/4(Torque_RLwc) -> Torque_RLwc/1
  VDC/6(Max_Torque_RL) -> Max_Torque_RL/1
  Accumulator Power/3(PowerMean500ms) -> PowerMean500ms/1
  VDC/8(Max_Fx_RL) -> Max_Fx_RL/1
  [RL_rads] -> Power limitation/4(Rev_L [rads])
  Constant17/1 -> Controls Temperature by limiting Torque/4(SoC_Low)
  If Action Subsystem/1(Motor_Tq_R) -> Merge/1
  VDC_Power_Limit/1 -> VDC/22(Limit_Power)
  Demux/4 -> TV_Flag_Power/1
  Calculate Current Conversion/1(Current R [A]) -> Merge2/2
  Pumps_Controller/1(Pumps_Control) -> Pumps_Control/1
  Current 0/2(Current R) -> Merge2/1
  [BrakeSensor_Value] -> Controls Temperature by limiting Torque/8(Brake_pedal)
  Abs3/1 -> Signal Conversion3/1, Signal Conversion2/1
  VDC/3(Torque_RRwc) -> Torque_RRwc/1
  Controls Temperature by limiting Torque/3(Accu_Temperature_Limitation_Flag) -> MATLAB Function1/1(Flag_Temp_Accu)
  VDC/16(SKF_act) -> SKF_actual/1
  [Motor_Tq_L] -> Controls Temperature by limiting Torque/7(Motor_Tq_L)
  VDC_Max_Regenerative_Torque/1 -> Transmission Gear Ratio/1
  Constant20/1 -> VDC/27(CKF_Initial)
  SteeringSensor/1 -> SteeringSensor_Value/1, VDC/5(Steer_An)
  Vel_RL_kmh/1 -> Abs1/1
  CriticalDisconnection/1 -> SAFETY BLOCK/3(CriticalDisconnection)
  If Action Subsystem/2(Motor_Tq_L) -> Merge3/1
  Gear Ratio/1 -> SoP selection and sum of max WHEEL Tq available/5(Gear_Ratio)
  RL_rads/1 -> Abs2/1
  [Temp_Cell] -> power_limitation1/3(max_cell_temp)
  [BrakeSensor_Value] -> SoP selection and sum of max WHEEL Tq available/4(Brake_Pedal)
  Controls Temperature by limiting Torque/1(Tq_R) -> Merge/2
  power_limitation1/3(Motors_Temperature_Limitation_Flag) -> MATLAB Function/3(Flag_Temp_Motor)
  Abs1/1 -> VDC/6(Velocity_RL_km/h)
  ACCEL_F_X_SI/1 -> VDC/16(Acceleration_X_Front)
  Constant18/1 -> [Apps_Sat_Down], VDC/19(APPS_Sat_Dwn)
  VDC_K_Reduction_Temperature/1 -> Terminator2/1
  Gain/1 -> Display3/1, [Motor_Tq_L]
  VDC_K_Reduction_P/1 -> Terminator1/1
  Merge/1 -> Display/1, Power limitation/1(Tq_R), Meas VDC Torque_R/1
  [Motor_Tq_R] -> Controls Temperature by limiting Torque/6(Motor_Tq_R)
  SAFETY BLOCK/3(Brake_Implausibility) -> Brake_Implausibility/1
  power_limitation1/5(SoP_Regen) -> SoP selection and sum of max WHEEL Tq available/2(SoP_Charge)
  If/2 -> Controls Temperature by limiting Torque/Action
  Calculate Current Conversion/2(Current L [A]) -> Merge1/2
  Gain1/1 -> Display2/1, [Motor_Tq_R]
  Merge3/1 -> Power limitation/2(Tq_L), Meas VDC Torque_L/1, Display1/1
  [APPS1_Value] -> SoP selection and sum of max WHEEL Tq available/3(Gas_Pedal)
  [Temp_Motors] -> Controls Temperature by limiting Torque/1(max_motor_temp)
  TV_Mode/1 -> [TV_mode], VDC/2(Failure_Contingency)
  power_limitation1/4(SoP_Discharge) -> SoP selection and sum of max WHEEL Tq available/1(SoP_Discharge)
  [APPS1_Value] -> VDC/3(APPS1_0_to_1)
  Car_State/1 -> [Car_State]
  SoP selection and sum of max WHEEL Tq available/1(Sum_wheel_Tq_max) -> VDC/31(Sum_Tq_max)
  Constant19/1 -> VDC/20(APPS_Sat_Up)
  Max Tq per motor [Nm]/1 -> SoP selection and sum of max WHEEL Tq available/6(Max_Tq_motor)
  Temp_IGBT/1 -> power_limitation1/2(max_inverter_temp), [Temp_IGBT]
  Merge1/1 -> Display6/1, current_L/1
  MATLAB Function1/1(Flag_Temp) -> Flag_Temp merged/1(Flag_Temp_else)
  Signal Conversion3/1 -> VDC/29(Velocity_RR_rad/s)
  Constant11/1 -> VDC/21(Max_Regen_Torque)
  Controls Temperature by limiting Torque/4(Inverters_Temperature_Limitation_Flag) -> MATLAB Function1/2(Flag_Temp_Inv)
  MATLAB Function/1(Flag_Temp_FM0) -> Flag_Temp merged/2(Flag_Temp_FM0)
  VDC/2(Torque_R_wheel) -> Gain1/1, Torque_R/1
  VDC/15(Regenetarive_EN) -> Regenerative_Enable/1
  VDC/1(Torque_L_wheel) -> Gain/1, Torque_L/1
  Merge2/1 -> Display5/1, current_R/1
  [Power_W] -> W to kW/1(Power)
  Controls Temperature by limiting Torque/2(Tq_L) -> Merge3/2
  Susp_F_L/1 -> VDC/8(Suspension_FL_N)
  W to kW/1(Out) -> VDC/12(Power_kW)
  APPS1_Value/1 -> [APPS1_Value], SAFETY BLOCK/6(APPS1_Value)
  Power limitation/2(Tq_L_lim) -> Calculate Current Conversion/2(Torque_L_motor)
  Constant/1 -> power_limitation1/4(SoC_Low)
  Susp_R_R/1 -> VDC/11(Suspension_RR_N)
  ShutdownClosed/1 -> SAFETY BLOCK/5(ShutdownClosed)
  Constant12/1 -> power_limitation1/5(SoC_High)
  If1/1 -> Calculate Current Conversion/Action
  [TV_mode] -> If/1
  Susp_F_R/1 -> VDC/9(Suspension_FR_N)
  VDC/9(Throttle) -> Throttle/1
  BrakeSensor_Value/1 -> [BrakeSensor_Value], SAFETY BLOCK/8(BrakeSensor_Value)
  SAFETY BLOCK/1(TorqueOK) -> Torque_OK/1, VDC/1(EnableVDC)
  Constant23/1 -> VDC/30(Yaw_Rate)
  Signal Conversion/1 -> VDC/28(Velocity_RL_rad/s)
  Constant9/1 -> Accumulator Power/1(TOTAL_V_BMS)
  [Car_State] -> Pumps_Controller/1(Car_State)
  ACCEL_R_Z_SI/1 -> VDC/15(Acceleration_Z_Rear)
  Accumulator Power/2(PowerLimitReached) -> PowerLimitReached/1
  Abs/1 -> VDC/7(Velocity_RR_km/h)
  ACCEL_R_Y_SI/1 -> VDC/14(Acceleration_Y_Rear)
  Demux/2 -> TV_Flag_WheelSpinRR/1
  TorqueEnable/1 -> SAFETY BLOCK/2(TorqueEnable)
  Demux/1 -> TV_Flag_CarBehaviour/1
  Constant10/1 -> Accumulator Power/2(CURRENT_BMS)
  ACCEL_R_X_SI/1 -> VDC/13(Acceleration_X_Rear)
  VDC/13(TV_Flags) -> Demux/1
  Susp_R_L/1 -> VDC/10(Suspension_RL_N)
  VDC/11(Mass) -> Mass/1
  [Temp_IGBT] -> Pumps_Controller/2(T_Max_IGBT)
  VDC/10(Fy_R) -> Fy_R/1
  VDC/12(Handling) -> Handling/1
  Demux/3 -> TV_Flag_WheelSpinRL/1
  Constant13/1 -> Controls Temperature by limiting Torque/5(SoC_High)
  ACCEL_F_Z_SI/1 -> VDC/18(Acceleration_Z_Front)
  VDC/7(Max_Fx_RR) -> Max_Fx_RR/1
  VDC/5(Max_Torque_RR) -> Max_Torque_RR/1
  If/1 -> If Action Subsystem/Action
  [Car_State] -> SAFETY BLOCK/4(Car_State)
  VDC/17(CKF_act) -> CKF_actual/1
  RR_rads/1 -> Abs3/1
  Abs2/1 -> Signal Conversion/1, Signal Conversion1/1
  Signal Conversion1/1 -> [RL_rads]
  Signal Conversion2/1 -> [RR_rads]
  Constant2/1 -> VDC/25(Cte_CKF)
  Constant3/1 -> VDC/24(Cte_SKF)

== system OPENXWD/CarMaker/IPG Vehicle/PowerTrain/Electric Powertrain/E-Gas // E-Motor/Subsystem/Accumulator Power ==
  TOTAL_V_BMS : Inport
  CURRENT_BMS : Inport  Port=2
  PowerLimitDetection : Subsystem  TreatAsAtomicUnit=on
  Product : Product
  AccumulatorPower [W] : Outport  VectorParamsAs1DForOutWhenUnconnected=off
  PowerLimitReached : Outport  Port=2  VectorParamsAs1DForOutWhenUnconnected=off
  PowerMean500ms : Outport  Port=3  VectorParamsAs1DForOutWhenUnconnected=off
  wires:
  Product/1 -> AccumulatorPower [W]/1, PowerLimitDetection/1(Power)
  PowerLimitDetection/1(PowerLimitReached) -> PowerLimitReached/1
  PowerLimitDetection/2(PowerMean500ms) -> PowerMean500ms/1
  TOTAL_V_BMS/1 -> Product/1
  CURRENT_BMS/1 -> Product/2

== system OPENXWD/CarMaker/IPG Vehicle/PowerTrain/Electric Powertrain/E-Gas // E-Motor/Subsystem/Calculate Current Conversion ==
  Torque_R_motor : Inport
  Torque_L_motor : Inport  Port=2
  Action Port : ActionPort  ActionPortLabel=if(u1 == 1)
  Gain : Gain  Gain=-1
  KT_L_TORKY : Subsystem  TreatAsAtomicUnit=on
  KT_R_EMY : Subsystem  TreatAsAtomicUnit=on
  Current R [A] : Outport  VectorParamsAs1DForOutWhenUnconnected=off
  Current L [A] : Outport  Port=2  VectorParamsAs1DForOutWhenUnconnected=off
  wires:
  Torque_R_motor/1 -> KT_R_EMY/1(Torque)
  Torque_L_motor/1 -> KT_L_TORKY/1(Torque)
  Gain/1 -> Current L [A]/1
  KT_R_EMY/1(Current) -> Current R [A]/1
  KT_L_TORKY/1(Current) -> Gain/1

== system OPENXWD/CarMaker/IPG Vehicle/PowerTrain/Electric Powertrain/E-Gas // E-Motor/Subsystem/Controls Temperature by limiting Torque ==
  note: Outputs:
      | Flags: 1 means power is being limited by temperature, 0 means not limited
      | SoP_discharge: State of Power for discharging
      | SoP_charge: State of Power for charging
  note: Inputs:
      | max_cell_temp: signal from AMS_Master (Highest_Cell_Temp) [ºC]
      | max_inverter_temp: highest temperature of any of the inverters [ºC]
      | max_motor_temp: highest temperature of any of the motors [ºC]
      | SoC_Low, SoC_High: Lowest & Highest cell state of charge (0-100) [%]
  max_motor_temp : Inport
  max_inverter_temp : Inport  Port=2
  max_cell_temp : Inport  Port=3
  SoC_Low : Inport  Port=4
  SoC_High : Inport  Port=5
  Motor_Tq_R : Inport  Port=6
  Motor_Tq_L : Inport  Port=7
  Brake_pedal : Inport  Port=8
  Action Port : ActionPort  ActionPortLabel=else
  Max_Tq_per_motor : Constant  Value=120
  Saturation : Saturate  UpperLimit=1  LowerLimit=0
  Saturation1 : Saturate  UpperLimit=1  LowerLimit=0
  SoC_SoP : Subsystem
  Tq_limitation because of Temp : MATLAB Function  TreatAsAtomicUnit=on
  initial_limitation : Constant  Value=0.4
  temperature_SoP : Subsystem
  Tq_R : Outport  VectorParamsAs1DForOutWhenUnconnected=off
  Tq_L : Outport  Port=2  VectorParamsAs1DForOutWhenUnconnected=off
  Accu_Temperature_Limitation_Flag : Outport  Port=3
  Inverters_Temperature_Limitation_Flag : Outport  Port=4
  Motors_Temperature_Limitation_Flag : Outport  Port=5
  wires:
  temperature_SoP/1(SoP) -> SoC_SoP/3(SoP_Temperature)  "temperature_SoP"
  SoC_Low/1 -> SoC_SoP/1(SoC_Low)
  Saturation1/1 -> Tq_limitation because of Temp/2(SoP_Charge)
  SoC_High/1 -> SoC_SoP/2(SoC_High)
  initial_limitation/1 -> temperature_SoP/4(initial_limitation)
  Saturation/1 -> Tq_limitation because of Temp/1(SoP_Discharge)
  temperature_SoP/4(Motors_Temperature_Limitation_Flag) -> Motors_Temperature_Limitation_Flag/1
  temperature_SoP/2(Accu_Temperature_Limitation_Flag) -> Accu_Temperature_Limitation_Flag/1
  SoC_SoP/2(SoP_Regen) -> Saturation1/1  "SoP_Regen"
  max_inverter_temp/1 -> temperature_SoP/2(max_inverter_temp)
  SoC_SoP/1(SoP_Discharge) -> Saturation/1  "SoP_Discharge"
  temperature_SoP/3(Inverters_Temperature_Limitation_Flag) -> Inverters_Temperature_Limitation_Flag/1
  max_cell_temp/1 -> temperature_SoP/3(max_cell_temp), SoC_SoP/4(max_cell_temp)
  max_motor_temp/1 -> temperature_SoP/1(max_motor_temp)
  Brake_pedal/1 -> Tq_limitation because of Temp/3(Brake_pedal)
  Motor_Tq_R/1 -> Tq_limitation because of Temp/4(Tq_R)
  Motor_Tq_L/1 -> Tq_limitation because of Temp/5(Tq_L)
  Tq_limitation because of Temp/1(Tq_R_limited) -> Tq_R/1
  Tq_limitation because of Temp/2(Tq_L_limited) -> Tq_L/1
  Max_Tq_per_motor/1 -> Tq_limitation because of Temp/6(Max_Tq_per_motor)

== system OPENXWD/CarMaker/IPG Vehicle/PowerTrain/Electric Powertrain/E-Gas // E-Motor/Subsystem/Current 0 ==
  Action Port : ActionPort  ActionPortLabel=else
  Constant : Constant  Value=0
  Constant1 : Constant  Value=0
  Current L : Outport  VectorParamsAs1DForOutWhenUnconnected=off
  Current R : Outport  Port=2  VectorParamsAs1DForOutWhenUnconnected=off
  wires:
  Constant/1 -> Current L/1
  Constant1/1 -> Current R/1

== system OPENXWD/CarMaker/IPG Vehicle/PowerTrain/Electric Powertrain/E-Gas // E-Motor/Subsystem/If Action Subsystem ==
  note: Tq already limited (because of Temp and Power) with the SoC
  In1 : Inport
  In2 : Inport  Port=2
  Action Port : ActionPort  ActionPortLabel=if(u1 == 0)
  Motor_Tq_R : Outport  VectorParamsAs1DForOutWhenUnconnected=off
  Motor_Tq_L : Outport  Port=2  VectorParamsAs1DForOutWhenUnconnected=off
  wires:
  In1/1 -> Motor_Tq_R/1
  In2/1 -> Motor_Tq_L/1

== system OPENXWD/CarMaker/IPG Vehicle/PowerTrain/Electric Powertrain/E-Gas // E-Motor/Subsystem/Power limitation ==
  Tq_R : Inport
  Tq_L : Inport  Port=2
  Rev_R [rads] : Inport  Port=3
  Rev_L [rads] : Inport  Port=4
  Braking : Inport  Port=5
  MATLAB Function : MATLAB Function  TreatAsAtomicUnit=on
  Max_Power_charge [kW] : Constant  Value=60
  Max_Power_discharge [kW] : Constant  Value=80
  Tq_R_lim : Outport  VectorParamsAs1DForOutWhenUnconnected=off
  Tq_L_lim : Outport  Port=2  VectorParamsAs1DForOutWhenUnconnected=off
  wires:
  Tq_R/1 -> MATLAB Function/1(Tq_R)
  Tq_L/1 -> MATLAB Function/2(Tq_L)
  Rev_R [rads]/1 -> MATLAB Function/3(Rev_R)
  Rev_L [rads]/1 -> MATLAB Function/4(Rev_L)
  Braking/1 -> MATLAB Function/5(Braking)
  Max_Power_discharge [kW]/1 -> MATLAB Function/6(Max_Power_Discharge)
  Max_Power_charge [kW]/1 -> MATLAB Function/7(Max_Power_Charge)
  MATLAB Function/1(Tq_R_lim) -> Tq_R_lim/1
  MATLAB Function/2(Tq_L_lim) -> Tq_L_lim/1

== system OPENXWD/CarMaker/IPG Vehicle/PowerTrain/Electric Powertrain/E-Gas // E-Motor/Subsystem/Pumps_Controller ==
  note: if car is in rtd or temperature of igbt is more than 50 degrees
  Car_State : Inport
  T_Max_IGBT : Inport  Port=2
  Compare To Constant : simulink/Logic and Bit Operations/Compare To Constant  relop=>  const=50  OutDataTypeStr=boolean
  Compare To Constant1 : simulink/Logic and Bit Operations/Compare To Constant  relop===  const=15  OutDataTypeStr=boolean
  DocBlock1 : simulink/Model-Wide Utilities/DocBlock  DocumentType=Text
      content=|
      | Aquest mòdul activa les bombes sempre que:
      | o bé s'està conduint
      | o bé la temperatura dels igbts de l'inversor supera 50 graus
  If : If  IfExpression=u1 == 1
  Logical Operator : Logic  Operator=OR  AllPortsSameDT=off  OutDataTypeStr=boolean
  Merge : Merge
  Pumps_Control_OFF : Subsystem  TreatAsAtomicUnit=on
  Pumps_Control_ON : Subsystem  TreatAsAtomicUnit=on
  Pumps_Control : Outport  VectorParamsAs1DForOutWhenUnconnected=off
  wires:
  Pumps_Control_OFF/1(0) -> Merge/2
  Car_State/1 -> Compare To Constant1/1
  If/2 -> Pumps_Control_OFF/Action
  If/1 -> Pumps_Control_ON/Action
  Pumps_Control_ON/1(1) -> Merge/1
  T_Max_IGBT/1 -> Compare To Constant/1
  Merge/1 -> Pumps_Control/1
  Logical Operator/1 -> If/1
  Compare To Constant/1 -> Logical Operator/2
  Compare To Constant1/1 -> Logical Operator/1

== system OPENXWD/CarMaker/IPG Vehicle/PowerTrain/Electric Powertrain/E-Gas // E-Motor/Subsystem/SAFETY BLOCK ==
  note: CriticalDisconnection -> 1
      | OK -> 0
  Power_W : Inport
  TorqueEnable : Inport  Port=2
  CriticalDisconnection : Inport  Port=3
  Car_State : Inport  Port=4
  ShutdownClosed : Inport  Port=5
  APPS1_Value : Inport  Port=6
  APPS2_Value : Inport  Port=7
  BrakeSensor_Value : Inport  Port=8
  APPS_IMPLAUSIBILITY : Subsystem
  BRAKE_IMPLAUSIBILITY : Subsystem
  Compare To Constant : simulink/Logic and Bit Operations/Compare To Constant  relop===  const=15  OutDataTypeStr=boolean
  Logical Operator : Logic  Inputs=6  OutDataTypeStr=boolean
  Logical Operator1 : Logic  Operator=NOT  IconShape=distinctive  AllPortsSameDT=off  OutDataTypeStr=boolean
  Logical Operator2 : Logic  Operator=NOT  IconShape=distinctive  AllPortsSameDT=off  OutDataTypeStr=boolean
  NOT : Logic  Operator=NOT  IconShape=distinctive  AllPortsSameDT=off  OutDataTypeStr=boolean
  "Power is under 80kW " : simulink/Logic and Bit Operations/Compare To Constant  relop=<  const=80000  OutDataTypeStr=boolean
  Terminator : Terminator
  TorqueOK : Outport  VectorParamsAs1DForOutWhenUnconnected=off
  APPS_Implausibility : Outport  Port=2  VectorParamsAs1DForOutWhenUnconnected=off
  Brake_Implausibility : Outport  Port=3  VectorParamsAs1DForOutWhenUnconnected=off
  wires:
  Logical Operator/1 -> TorqueOK/1
  ShutdownClosed/1 -> Logical Operator/1
  Car_State/1 -> Compare To Constant/1
  NOT/1 -> Logical Operator/3
  CriticalDisconnection/1 -> NOT/1
  TorqueEnable/1 -> Logical Operator/2
  Power_W/1 -> "Power is under 80kW "/1
  BrakeSensor_Value/1 -> BRAKE_IMPLAUSIBILITY/3(BrakeSensor_Value)
  APPS2_Value/1 -> BRAKE_IMPLAUSIBILITY/2(APPS2_Value), APPS_IMPLAUSIBILITY/2(APPS2)
  APPS1_Value/1 -> BRAKE_IMPLAUSIBILITY/1(APPS1_Value), APPS_IMPLAUSIBILITY/1(APPS1)
  BRAKE_IMPLAUSIBILITY/1(OK_BRS) -> Logical Operator/6, Logical Operator2/1
  Logical Operator2/1 -> Brake_Implausibility/1
  Logical Operator1/1 -> APPS_Implausibility/1
  Compare To Constant/1 -> Logical Operator/4
  APPS_IMPLAUSIBILITY/1(OK) -> Logical Operator/5, Logical Operator1/1
  "Power is under 80kW "/1 -> Terminator/1
